simulink model "Servo_Motor"  (R2025b)
settings: Solver=VariableStepAuto  StartTime=0.0  StopTime=10.0  RelTol=1e-3
model workspace (MAT data in the model file):
  J = 5e-05
  K = 0.2
  L = 0.001
  R = 4
  Ts = 0.01
  V = 7.4
  b = 0.0005
  ki = 7.33
  kp = 9.39

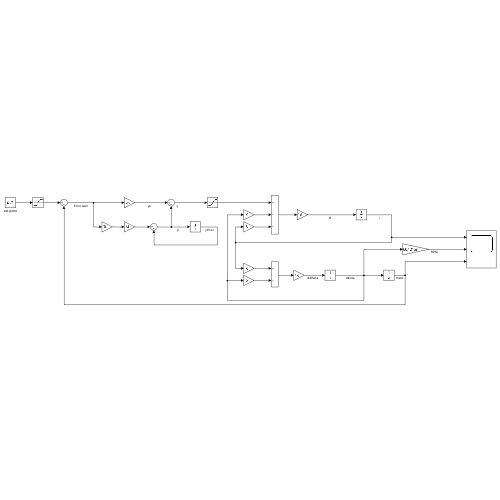
[thumbnail: Simulink's stored preview of the top-level diagram]
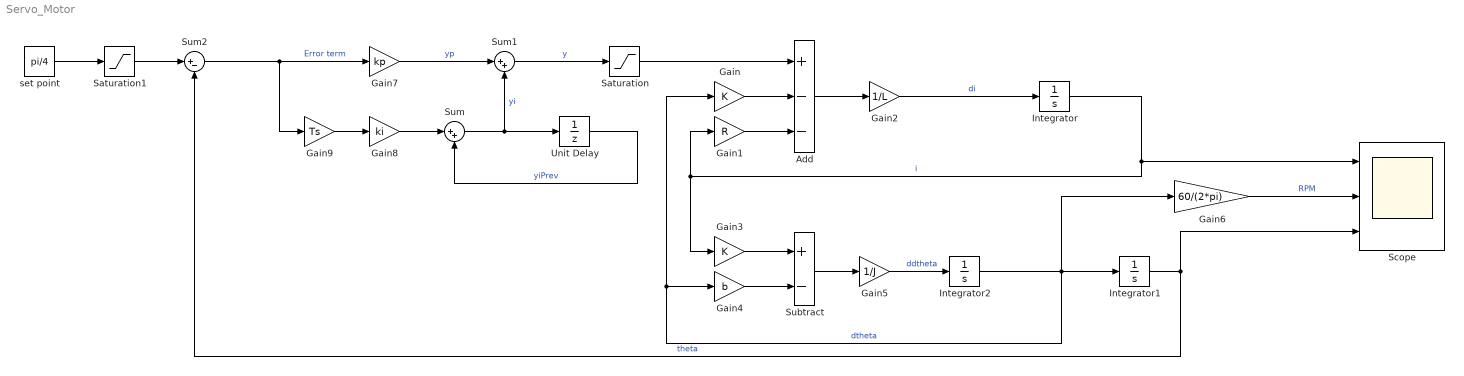
== system Servo_Motor ==
  Add : Sum  Inputs=+--
  Gain : Gain  Gain=K
  Gain1 : Gain  Gain=R
  Gain2 : Gain  Gain=1/L
  Gain3 : Gain  Gain=K
  Gain4 : Gain  Gain=b
  Gain5 : Gain  Gain=1/J
  Gain6 : Gain  Gain=60/(2*pi)
  Gain7 : Gain  Gain=kp
  Gain8 : Gain  Gain=ki
  Gain9 : Gain  Gain=Ts
  Integrator : Integrator
  Integrator1 : Integrator
  Integrator2 : Integrator
  Saturation : Saturate  UpperLimit=V  LowerLimit=-V
  Saturation1 : Saturate  UpperLimit=pi/4  LowerLimit=-pi/4
  Scope : Scope  NumInputPorts=3
      settings: ActiveDisplayYMinimum=-0.43284807398949154  ActiveDisplayYMaximum=1.8763225568429218
  Subtract : Sum  Inputs=+-
  Sum : Sum  Inputs=|++
  Sum1 : Sum  Inputs=|++
  Sum2 : Sum  Inputs=|+-
  Unit Delay : UnitDelay  InitialCondition=1  SampleTime=Ts  HasFrameUpgradeWarning=on
  set point : Constant  Value=pi/4
  wires:
  Gain2/1 -> Integrator/1  "di"
  Integrator/1 -> Gain1/1, Gain3/1, Scope/1  "i"
  Integrator2/1 -> Gain6/1, Gain4/1, Gain/1, Integrator1/1  "dtheta"
  Integrator1/1 -> Scope/3, Sum2/2  "theta"
  Gain5/1 -> Integrator2/1  "ddtheta"
  Gain/1 -> Add/2
  Gain1/1 -> Add/3
  Add/1 -> Gain2/1
  Gain3/1 -> Subtract/1
  Gain4/1 -> Subtract/2
  Subtract/1 -> Gain5/1
  Gain6/1 -> Scope/2  "RPM"
  Gain8/1 -> Sum/1
  Gain9/1 -> Gain8/1
  Sum1/1 -> Saturation/1  "y"
  Gain7/1 -> Sum1/1  "yp"
  Unit Delay/1 -> Sum/2  "yiPrev"
  Sum/1 -> Unit Delay/1, Sum1/2  "yi"
  set point/1 -> Saturation1/1
  Sum2/1 -> Gain9/1, Gain7/1  "Error term"
  Saturation/1 -> Add/1
  Saturation1/1 -> Sum2/1
